simulink model "TST_AirHt_Ctl"  (R2016b)
settings: Solver=FixedStepDiscrete  StartTime=0.0  StopTime=simTime  FixedStep=sampleTime  RelTol=1e-3
values from neighbouring files (symbols this model uses):
  testCase = 1    [initTST_AirHt_Ctl_001.m]    (also in initTST_AirHt_Ctl_002.m = 2; initTST_AirHt_Ctl_003.m = 3; initTST_AirHt_Ctl_004.m = 4; initTST_AirHt_Ctl_005.m = 5)
libraries: simulink x53, UnitTest_Lib x26
(part 3 of 4)

== system TST_AirHt_Ctl/simulationInput/testSignals_R006 ==
  BC : BusCreator  Inputs=21
  spec_AirHt_st : FromWorkspace  VariableName=testSig_AirHt_st  Interpolate=off  OutputAfterFinalValue=Holding final value
  spec_Air_tAFS_mp : FromWorkspace  VariableName=testSig_Air_tAFS_mp  Interpolate=off  OutputAfterFinalValue=Holding final value
  spec_Air_tCACDs_mp : FromWorkspace  VariableName=testSig_Air_tCACDs_mp  Interpolate=off  OutputAfterFinalValue=Holding final value
  spec_Air_tIntkVUs : FromWorkspace  VariableName=testSig_Air_tIntkVUs  Interpolate=off  OutputAfterFinalValue=Holding final value
  spec_BattU_u : FromWorkspace  VariableName=testSig_BattU_u  Interpolate=off  OutputAfterFinalValue=Holding final value
  spec_CEngDsT_t : FromWorkspace  VariableName=testSig_CEngDsT_t  Interpolate=off  OutputAfterFinalValue=Holding final value
  spec_CoEng_st : FromWorkspace  VariableName=testSig_CoEng_st  Interpolate=off  OutputAfterFinalValue=Holding final value
  spec_DSM_bAirHtAFST : FromWorkspace  VariableName=testSig_DSM_bAirHtAFST  Interpolate=off  OutputAfterFinalValue=Holding final value
  spec_DSM_bAirHtCACDs : FromWorkspace  VariableName=testSig_DSM_bAirHtCACDs  Interpolate=off  OutputAfterFinalValue=Holding final value
  spec_DSM_bAirHtCEngDsT : FromWorkspace  VariableName=testSig_DSM_bAirHtCEngDsT  Interpolate=off  OutputAfterFinalValue=Holding final value
  spec_DSM_bAirHtEnvT : FromWorkspace  VariableName=testSig_DSM_bAirHtEnvT  Interpolate=off  OutputAfterFinalValue=Holding final value
  spec_DSM_bAirHtFuelT : FromWorkspace  VariableName=testSig_DSM_bAirHtFuelT  Interpolate=off  OutputAfterFinalValue=Holding final value
  spec_DSM_bAirHtIntkVUsT : FromWorkspace  VariableName=testSig_DSM_bAirHtIntkVUsT  Interpolate=off  OutputAfterFinalValue=Holding final value
  spec_DSM_bAirHtOilT : FromWorkspace  VariableName=testSig_DSM_bAirHtOilT  Interpolate=off  OutputAfterFinalValue=Holding final value
  spec_EnvT_t : FromWorkspace  VariableName=testSig_EnvT_t  Interpolate=off  OutputAfterFinalValue=Holding final value
  spec_Epm_nEng : FromWorkspace  VariableName=testSig_Epm_nEng  Interpolate=off  OutputAfterFinalValue=Holding final value
  spec_FuelT_t : FromWorkspace  VariableName=testSig_FuelT_t  Interpolate=off  OutputAfterFinalValue=Holding final value
  spec_GlwLmp_st : FromWorkspace  VariableName=testSig_GlwLmp_st  Interpolate=off  OutputAfterFinalValue=Holding final value
  spec_IAirHt_st : FromWorkspace  VariableName=testSig_IAirHt_st  Interpolate=off  OutputAfterFinalValue=Holding final value
  spec_Oil_tSwmp : FromWorkspace  VariableName=testSig_Oil_tSwmp  Interpolate=off  OutputAfterFinalValue=Holding final value
  spec_T15_st : FromWorkspace  VariableName=testSig_T15_st  Interpolate=off  OutputAfterFinalValue=Holding final value
  testSignals : Outport
  wires:
  BC/1 -> testSignals/1
  spec_T15_st/1 -> BC/1  "testSig_T15_st"
  spec_CoEng_st/1 -> BC/2  "testSig_CoEng_st"
  spec_Epm_nEng/1 -> BC/3  "testSig_Epm_nEng"
  spec_BattU_u/1 -> BC/4  "testSig_BattU_u"
  spec_CEngDsT_t/1 -> BC/5  "testSig_CEngDsT_t"
  spec_FuelT_t/1 -> BC/6  "testSig_FuelT_t"
  spec_Oil_tSwmp/1 -> BC/7  "testSig_Oil_tSwmp"
  spec_Air_tCACDs_mp/1 -> BC/8  "testSig_Air_tCACDs_mp"
  spec_Air_tAFS_mp/1 -> BC/9  "testSig_Air_tAFS_mp"
  spec_EnvT_t/1 -> BC/10  "testSig_EnvT_t"
  spec_Air_tIntkVUs/1 -> BC/11  "testSig_Air_tIntkVUs"
  spec_DSM_bAirHtCEngDsT/1 -> BC/12  "testSig_DSM_bAirHtCEngDsT"
  spec_DSM_bAirHtFuelT/1 -> BC/13  "testSig_DSM_bAirHtFuelT"
  spec_DSM_bAirHtOilT/1 -> BC/14  "testSig_DSM_bAirHtOilT"
  spec_DSM_bAirHtEnvT/1 -> BC/15  "testSig_DSM_bAirHtEnvT"
  spec_DSM_bAirHtCACDs/1 -> BC/16  "testSig_DSM_bAirHtCACDs"
  spec_DSM_bAirHtAFST/1 -> BC/17  "testSig_DSM_bAirHtAFST"
  spec_DSM_bAirHtIntkVUsT/1 -> BC/18  "testSig_DSM_bAirHtIntkVUsT"
  spec_AirHt_st/1 -> BC/19  "testSig_AirHt_st"
  spec_IAirHt_st/1 -> BC/20  "testSig_IAirHt_st"
  spec_GlwLmp_st/1 -> BC/21  "testSig_GlwLmp_st"

== system TST_AirHt_Ctl/simulationInput/testSignals_R007 ==
  BC : BusCreator  Inputs=21
  spec_AirHt_st : FromWorkspace  VariableName=testSig_AirHt_st  Interpolate=off  OutputAfterFinalValue=Holding final value
  spec_Air_tAFS_mp : FromWorkspace  VariableName=testSig_Air_tAFS_mp  Interpolate=off  OutputAfterFinalValue=Holding final value
  spec_Air_tCACDs_mp : FromWorkspace  VariableName=testSig_Air_tCACDs_mp  Interpolate=off  OutputAfterFinalValue=Holding final value
  spec_Air_tIntkVUs : FromWorkspace  VariableName=testSig_Air_tIntkVUs  Interpolate=off  OutputAfterFinalValue=Holding final value
  spec_BattU_u : FromWorkspace  VariableName=testSig_BattU_u  Interpolate=off  OutputAfterFinalValue=Holding final value
  spec_CEngDsT_t : FromWorkspace  VariableName=testSig_CEngDsT_t  Interpolate=off  OutputAfterFinalValue=Holding final value
  spec_CoEng_st : FromWorkspace  VariableName=testSig_CoEng_st  Interpolate=off  OutputAfterFinalValue=Holding final value
  spec_DSM_bAirHtAFST : FromWorkspace  VariableName=testSig_DSM_bAirHtAFST  Interpolate=off  OutputAfterFinalValue=Holding final value
  spec_DSM_bAirHtCACDs : FromWorkspace  VariableName=testSig_DSM_bAirHtCACDs  Interpolate=off  OutputAfterFinalValue=Holding final value
  spec_DSM_bAirHtCEngDsT : FromWorkspace  VariableName=testSig_DSM_bAirHtCEngDsT  Interpolate=off  OutputAfterFinalValue=Holding final value
  spec_DSM_bAirHtEnvT : FromWorkspace  VariableName=testSig_DSM_bAirHtEnvT  Interpolate=off  OutputAfterFinalValue=Holding final value
  spec_DSM_bAirHtFuelT : FromWorkspace  VariableName=testSig_DSM_bAirHtFuelT  Interpolate=off  OutputAfterFinalValue=Holding final value
  spec_DSM_bAirHtIntkVUsT : FromWorkspace  VariableName=testSig_DSM_bAirHtIntkVUsT  Interpolate=off  OutputAfterFinalValue=Holding final value
  spec_DSM_bAirHtOilT : FromWorkspace  VariableName=testSig_DSM_bAirHtOilT  Interpolate=off  OutputAfterFinalValue=Holding final value
  spec_EnvT_t : FromWorkspace  VariableName=testSig_EnvT_t  Interpolate=off  OutputAfterFinalValue=Holding final value
  spec_Epm_nEng : FromWorkspace  VariableName=testSig_Epm_nEng  Interpolate=off  OutputAfterFinalValue=Holding final value
  spec_FuelT_t : FromWorkspace  VariableName=testSig_FuelT_t  Interpolate=off  OutputAfterFinalValue=Holding final value
  spec_GlwLmp_st : FromWorkspace  VariableName=testSig_GlwLmp_st  Interpolate=off  OutputAfterFinalValue=Holding final value
  spec_IAirHt_st : FromWorkspace  VariableName=testSig_IAirHt_st  Interpolate=off  OutputAfterFinalValue=Holding final value
  spec_Oil_tSwmp : FromWorkspace  VariableName=testSig_Oil_tSwmp  Interpolate=off  OutputAfterFinalValue=Holding final value
  spec_T15_st : FromWorkspace  VariableName=testSig_T15_st  Interpolate=off  OutputAfterFinalValue=Holding final value
  testSignals : Outport
  wires:
  BC/1 -> testSignals/1
  spec_T15_st/1 -> BC/1  "testSig_T15_st"
  spec_CoEng_st/1 -> BC/2  "testSig_CoEng_st"
  spec_Epm_nEng/1 -> BC/3  "testSig_Epm_nEng"
  spec_BattU_u/1 -> BC/4  "testSig_BattU_u"
  spec_CEngDsT_t/1 -> BC/5  "testSig_CEngDsT_t"
  spec_FuelT_t/1 -> BC/6  "testSig_FuelT_t"
  spec_Oil_tSwmp/1 -> BC/7  "testSig_Oil_tSwmp"
  spec_Air_tCACDs_mp/1 -> BC/8  "testSig_Air_tCACDs_mp"
  spec_Air_tAFS_mp/1 -> BC/9  "testSig_Air_tAFS_mp"
  spec_EnvT_t/1 -> BC/10  "testSig_EnvT_t"
  spec_Air_tIntkVUs/1 -> BC/11  "testSig_Air_tIntkVUs"
  spec_DSM_bAirHtCEngDsT/1 -> BC/12  "testSig_DSM_bAirHtCEngDsT"
  spec_DSM_bAirHtFuelT/1 -> BC/13  "testSig_DSM_bAirHtFuelT"
  spec_DSM_bAirHtOilT/1 -> BC/14  "testSig_DSM_bAirHtOilT"
  spec_DSM_bAirHtEnvT/1 -> BC/15  "testSig_DSM_bAirHtEnvT"
  spec_DSM_bAirHtCACDs/1 -> BC/16  "testSig_DSM_bAirHtCACDs"
  spec_DSM_bAirHtAFST/1 -> BC/17  "testSig_DSM_bAirHtAFST"
  spec_DSM_bAirHtIntkVUsT/1 -> BC/18  "testSig_DSM_bAirHtIntkVUsT"
  spec_AirHt_st/1 -> BC/19  "testSig_AirHt_st"
  spec_IAirHt_st/1 -> BC/20  "testSig_IAirHt_st"
  spec_GlwLmp_st/1 -> BC/21  "testSig_GlwLmp_st"

== system TST_AirHt_Ctl/simulationInput/testSignals_R008 ==
  BC : BusCreator  Inputs=21
  spec_AirHt_st : FromWorkspace  VariableName=testSig_AirHt_st  Interpolate=off  OutputAfterFinalValue=Holding final value
  spec_Air_tAFS_mp : FromWorkspace  VariableName=testSig_Air_tAFS_mp  Interpolate=off  OutputAfterFinalValue=Holding final value
  spec_Air_tCACDs_mp : FromWorkspace  VariableName=testSig_Air_tCACDs_mp  Interpolate=off  OutputAfterFinalValue=Holding final value
  spec_Air_tIntkVUs : FromWorkspace  VariableName=testSig_Air_tIntkVUs  Interpolate=off  OutputAfterFinalValue=Holding final value
  spec_BattU_u : FromWorkspace  VariableName=testSig_BattU_u  Interpolate=off  OutputAfterFinalValue=Holding final value
  spec_CEngDsT_t : FromWorkspace  VariableName=testSig_CEngDsT_t  Interpolate=off  OutputAfterFinalValue=Holding final value
  spec_CoEng_st : FromWorkspace  VariableName=testSig_CoEng_st  Interpolate=off  OutputAfterFinalValue=Holding final value
  spec_DSM_bAirHtAFST : FromWorkspace  VariableName=testSig_DSM_bAirHtAFST  Interpolate=off  OutputAfterFinalValue=Holding final value
  spec_DSM_bAirHtCACDs : FromWorkspace  VariableName=testSig_DSM_bAirHtCACDs  Interpolate=off  OutputAfterFinalValue=Holding final value
  spec_DSM_bAirHtCEngDsT : FromWorkspace  VariableName=testSig_DSM_bAirHtCEngDsT  Interpolate=off  OutputAfterFinalValue=Holding final value
  spec_DSM_bAirHtEnvT : FromWorkspace  VariableName=testSig_DSM_bAirHtEnvT  Interpolate=off  OutputAfterFinalValue=Holding final value
  spec_DSM_bAirHtFuelT : FromWorkspace  VariableName=testSig_DSM_bAirHtFuelT  Interpolate=off  OutputAfterFinalValue=Holding final value
  spec_DSM_bAirHtIntkVUsT : FromWorkspace  VariableName=testSig_DSM_bAirHtIntkVUsT  Interpolate=off  OutputAfterFinalValue=Holding final value
  spec_DSM_bAirHtOilT : FromWorkspace  VariableName=testSig_DSM_bAirHtOilT  Interpolate=off  OutputAfterFinalValue=Holding final value
  spec_EnvT_t : FromWorkspace  VariableName=testSig_EnvT_t  Interpolate=off  OutputAfterFinalValue=Holding final value
  spec_Epm_nEng : FromWorkspace  VariableName=testSig_Epm_nEng  Interpolate=off  OutputAfterFinalValue=Holding final value
  spec_FuelT_t : FromWorkspace  VariableName=testSig_FuelT_t  Interpolate=off  OutputAfterFinalValue=Holding final value
  spec_GlwLmp_st : FromWorkspace  VariableName=testSig_GlwLmp_st  Interpolate=off  OutputAfterFinalValue=Holding final value
  spec_IAirHt_st : FromWorkspace  VariableName=testSig_IAirHt_st  Interpolate=off  OutputAfterFinalValue=Holding final value
  spec_Oil_tSwmp : FromWorkspace  VariableName=testSig_Oil_tSwmp  Interpolate=off  OutputAfterFinalValue=Holding final value
  spec_T15_st : FromWorkspace  VariableName=testSig_T15_st  Interpolate=off  OutputAfterFinalValue=Holding final value
  testSignals : Outport
  wires:
  BC/1 -> testSignals/1
  spec_T15_st/1 -> BC/1  "testSig_T15_st"
  spec_CoEng_st/1 -> BC/2  "testSig_CoEng_st"
  spec_Epm_nEng/1 -> BC/3  "testSig_Epm_nEng"
  spec_BattU_u/1 -> BC/4  "testSig_BattU_u"
  spec_CEngDsT_t/1 -> BC/5  "testSig_CEngDsT_t"
  spec_FuelT_t/1 -> BC/6  "testSig_FuelT_t"
  spec_Oil_tSwmp/1 -> BC/7  "testSig_Oil_tSwmp"
  spec_Air_tCACDs_mp/1 -> BC/8  "testSig_Air_tCACDs_mp"
  spec_Air_tAFS_mp/1 -> BC/9  "testSig_Air_tAFS_mp"
  spec_EnvT_t/1 -> BC/10  "testSig_EnvT_t"
  spec_Air_tIntkVUs/1 -> BC/11  "testSig_Air_tIntkVUs"
  spec_DSM_bAirHtCEngDsT/1 -> BC/12  "testSig_DSM_bAirHtCEngDsT"
  spec_DSM_bAirHtFuelT/1 -> BC/13  "testSig_DSM_bAirHtFuelT"
  spec_DSM_bAirHtOilT/1 -> BC/14  "testSig_DSM_bAirHtOilT"
  spec_DSM_bAirHtEnvT/1 -> BC/15  "testSig_DSM_bAirHtEnvT"
  spec_DSM_bAirHtCACDs/1 -> BC/16  "testSig_DSM_bAirHtCACDs"
  spec_DSM_bAirHtAFST/1 -> BC/17  "testSig_DSM_bAirHtAFST"
  spec_DSM_bAirHtIntkVUsT/1 -> BC/18  "testSig_DSM_bAirHtIntkVUsT"
  spec_AirHt_st/1 -> BC/19  "testSig_AirHt_st"
  spec_IAirHt_st/1 -> BC/20  "testSig_IAirHt_st"
  spec_GlwLmp_st/1 -> BC/21  "testSig_GlwLmp_st"

== system TST_AirHt_Ctl/simulationInput/testSignals_R009 ==
  BC : BusCreator  Inputs=21
  spec_AirHt_st : FromWorkspace  VariableName=testSig_AirHt_st  Interpolate=off  OutputAfterFinalValue=Holding final value
  spec_Air_tAFS_mp : FromWorkspace  VariableName=testSig_Air_tAFS_mp  Interpolate=off  OutputAfterFinalValue=Holding final value
  spec_Air_tCACDs_mp : FromWorkspace  VariableName=testSig_Air_tCACDs_mp  Interpolate=off  OutputAfterFinalValue=Holding final value
  spec_Air_tIntkVUs : FromWorkspace  VariableName=testSig_Air_tIntkVUs  Interpolate=off  OutputAfterFinalValue=Holding final value
  spec_BattU_u : FromWorkspace  VariableName=testSig_BattU_u  Interpolate=off  OutputAfterFinalValue=Holding final value
  spec_CEngDsT_t : FromWorkspace  VariableName=testSig_CEngDsT_t  Interpolate=off  OutputAfterFinalValue=Holding final value
  spec_CoEng_st : FromWorkspace  VariableName=testSig_CoEng_st  Interpolate=off  OutputAfterFinalValue=Holding final value
  spec_DSM_bAirHtAFST : FromWorkspace  VariableName=testSig_DSM_bAirHtAFST  Interpolate=off  OutputAfterFinalValue=Holding final value
  spec_DSM_bAirHtCACDs : FromWorkspace  VariableName=testSig_DSM_bAirHtCACDs  Interpolate=off  OutputAfterFinalValue=Holding final value
  spec_DSM_bAirHtCEngDsT : FromWorkspace  VariableName=testSig_DSM_bAirHtCEngDsT  Interpolate=off  OutputAfterFinalValue=Holding final value
  spec_DSM_bAirHtEnvT : FromWorkspace  VariableName=testSig_DSM_bAirHtEnvT  Interpolate=off  OutputAfterFinalValue=Holding final value
  spec_DSM_bAirHtFuelT : FromWorkspace  VariableName=testSig_DSM_bAirHtFuelT  Interpolate=off  OutputAfterFinalValue=Holding final value
  spec_DSM_bAirHtIntkVUsT : FromWorkspace  VariableName=testSig_DSM_bAirHtIntkVUsT  Interpolate=off  OutputAfterFinalValue=Holding final value
  spec_DSM_bAirHtOilT : FromWorkspace  VariableName=testSig_DSM_bAirHtOilT  Interpolate=off  OutputAfterFinalValue=Holding final value
  spec_EnvT_t : FromWorkspace  VariableName=testSig_EnvT_t  Interpolate=off  OutputAfterFinalValue=Holding final value
  spec_Epm_nEng : FromWorkspace  VariableName=testSig_Epm_nEng  Interpolate=off  OutputAfterFinalValue=Holding final value
  spec_FuelT_t : FromWorkspace  VariableName=testSig_FuelT_t  Interpolate=off  OutputAfterFinalValue=Holding final value
  spec_GlwLmp_st : FromWorkspace  VariableName=testSig_GlwLmp_st  Interpolate=off  OutputAfterFinalValue=Holding final value
  spec_IAirHt_st : FromWorkspace  VariableName=testSig_IAirHt_st  Interpolate=off  OutputAfterFinalValue=Holding final value
  spec_Oil_tSwmp : FromWorkspace  VariableName=testSig_Oil_tSwmp  Interpolate=off  OutputAfterFinalValue=Holding final value
  spec_T15_st : FromWorkspace  VariableName=testSig_T15_st  Interpolate=off  OutputAfterFinalValue=Holding final value
  testSignals : Outport
  wires:
  BC/1 -> testSignals/1
  spec_T15_st/1 -> BC/1  "testSig_T15_st"
  spec_CoEng_st/1 -> BC/2  "testSig_CoEng_st"
  spec_Epm_nEng/1 -> BC/3  "testSig_Epm_nEng"
  spec_BattU_u/1 -> BC/4  "testSig_BattU_u"
  spec_CEngDsT_t/1 -> BC/5  "testSig_CEngDsT_t"
  spec_FuelT_t/1 -> BC/6  "testSig_FuelT_t"
  spec_Oil_tSwmp/1 -> BC/7  "testSig_Oil_tSwmp"
  spec_Air_tCACDs_mp/1 -> BC/8  "testSig_Air_tCACDs_mp"
  spec_Air_tAFS_mp/1 -> BC/9  "testSig_Air_tAFS_mp"
  spec_EnvT_t/1 -> BC/10  "testSig_EnvT_t"
  spec_Air_tIntkVUs/1 -> BC/11  "testSig_Air_tIntkVUs"
  spec_DSM_bAirHtCEngDsT/1 -> BC/12  "testSig_DSM_bAirHtCEngDsT"
  spec_DSM_bAirHtFuelT/1 -> BC/13  "testSig_DSM_bAirHtFuelT"
  spec_DSM_bAirHtOilT/1 -> BC/14  "testSig_DSM_bAirHtOilT"
  spec_DSM_bAirHtEnvT/1 -> BC/15  "testSig_DSM_bAirHtEnvT"
  spec_DSM_bAirHtCACDs/1 -> BC/16  "testSig_DSM_bAirHtCACDs"
  spec_DSM_bAirHtAFST/1 -> BC/17  "testSig_DSM_bAirHtAFST"
  spec_DSM_bAirHtIntkVUsT/1 -> BC/18  "testSig_DSM_bAirHtIntkVUsT"
  spec_AirHt_st/1 -> BC/19  "testSig_AirHt_st"
  spec_IAirHt_st/1 -> BC/20  "testSig_IAirHt_st"
  spec_GlwLmp_st/1 -> BC/21  "testSig_GlwLmp_st"

== system TST_AirHt_Ctl/simulationInput/testSignals_R010 ==
  BC : BusCreator  Inputs=21
  spec_AirHt_st : FromWorkspace  VariableName=testSig_AirHt_st  Interpolate=off  OutputAfterFinalValue=Holding final value
  spec_Air_tAFS_mp : FromWorkspace  VariableName=testSig_Air_tAFS_mp  Interpolate=off  OutputAfterFinalValue=Holding final value
  spec_Air_tCACDs_mp : FromWorkspace  VariableName=testSig_Air_tCACDs_mp  Interpolate=off  OutputAfterFinalValue=Holding final value
  spec_Air_tIntkVUs : FromWorkspace  VariableName=testSig_Air_tIntkVUs  Interpolate=off  OutputAfterFinalValue=Holding final value
  spec_BattU_u : FromWorkspace  VariableName=testSig_BattU_u  Interpolate=off  OutputAfterFinalValue=Holding final value
  spec_CEngDsT_t : FromWorkspace  VariableName=testSig_CEngDsT_t  Interpolate=off  OutputAfterFinalValue=Holding final value
  spec_CoEng_st : FromWorkspace  VariableName=testSig_CoEng_st  Interpolate=off  OutputAfterFinalValue=Holding final value
  spec_DSM_bAirHtAFST : FromWorkspace  VariableName=testSig_DSM_bAirHtAFST  Interpolate=off  OutputAfterFinalValue=Holding final value
  spec_DSM_bAirHtCACDs : FromWorkspace  VariableName=testSig_DSM_bAirHtCACDs  Interpolate=off  OutputAfterFinalValue=Holding final value
  spec_DSM_bAirHtCEngDsT : FromWorkspace  VariableName=testSig_DSM_bAirHtCEngDsT  Interpolate=off  OutputAfterFinalValue=Holding final value
  spec_DSM_bAirHtEnvT : FromWorkspace  VariableName=testSig_DSM_bAirHtEnvT  Interpolate=off  OutputAfterFinalValue=Holding final value
  spec_DSM_bAirHtFuelT : FromWorkspace  VariableName=testSig_DSM_bAirHtFuelT  Interpolate=off  OutputAfterFinalValue=Holding final value
  spec_DSM_bAirHtIntkVUsT : FromWorkspace  VariableName=testSig_DSM_bAirHtIntkVUsT  Interpolate=off  OutputAfterFinalValue=Holding final value
  spec_DSM_bAirHtOilT : FromWorkspace  VariableName=testSig_DSM_bAirHtOilT  Interpolate=off  OutputAfterFinalValue=Holding final value
  spec_EnvT_t : FromWorkspace  VariableName=testSig_EnvT_t  Interpolate=off  OutputAfterFinalValue=Holding final value
  spec_Epm_nEng : FromWorkspace  VariableName=testSig_Epm_nEng  Interpolate=off  OutputAfterFinalValue=Holding final value
  spec_FuelT_t : FromWorkspace  VariableName=testSig_FuelT_t  Interpolate=off  OutputAfterFinalValue=Holding final value
  spec_GlwLmp_st : FromWorkspace  VariableName=testSig_GlwLmp_st  Interpolate=off  OutputAfterFinalValue=Holding final value
  spec_IAirHt_st : FromWorkspace  VariableName=testSig_IAirHt_st  Interpolate=off  OutputAfterFinalValue=Holding final value
  spec_Oil_tSwmp : FromWorkspace  VariableName=testSig_Oil_tSwmp  Interpolate=off  OutputAfterFinalValue=Holding final value
  spec_T15_st : FromWorkspace  VariableName=testSig_T15_st  Interpolate=off  OutputAfterFinalValue=Holding final value
  testSignals : Outport
  wires:
  BC/1 -> testSignals/1
  spec_T15_st/1 -> BC/1  "testSig_T15_st"
  spec_CoEng_st/1 -> BC/2  "testSig_CoEng_st"
  spec_Epm_nEng/1 -> BC/3  "testSig_Epm_nEng"
  spec_BattU_u/1 -> BC/4  "testSig_BattU_u"
  spec_CEngDsT_t/1 -> BC/5  "testSig_CEngDsT_t"
  spec_FuelT_t/1 -> BC/6  "testSig_FuelT_t"
  spec_Oil_tSwmp/1 -> BC/7  "testSig_Oil_tSwmp"
  spec_Air_tCACDs_mp/1 -> BC/8  "testSig_Air_tCACDs_mp"
  spec_Air_tAFS_mp/1 -> BC/9  "testSig_Air_tAFS_mp"
  spec_EnvT_t/1 -> BC/10  "testSig_EnvT_t"
  spec_Air_tIntkVUs/1 -> BC/11  "testSig_Air_tIntkVUs"
  spec_DSM_bAirHtCEngDsT/1 -> BC/12  "testSig_DSM_bAirHtCEngDsT"
  spec_DSM_bAirHtFuelT/1 -> BC/13  "testSig_DSM_bAirHtFuelT"
  spec_DSM_bAirHtOilT/1 -> BC/14  "testSig_DSM_bAirHtOilT"
  spec_DSM_bAirHtEnvT/1 -> BC/15  "testSig_DSM_bAirHtEnvT"
  spec_DSM_bAirHtCACDs/1 -> BC/16  "testSig_DSM_bAirHtCACDs"
  spec_DSM_bAirHtAFST/1 -> BC/17  "testSig_DSM_bAirHtAFST"
  spec_DSM_bAirHtIntkVUsT/1 -> BC/18  "testSig_DSM_bAirHtIntkVUsT"
  spec_AirHt_st/1 -> BC/19  "testSig_AirHt_st"
  spec_IAirHt_st/1 -> BC/20  "testSig_IAirHt_st"
  spec_GlwLmp_st/1 -> BC/21  "testSig_GlwLmp_st"

== system TST_AirHt_Ctl/simulationInput/testSignals_R011 ==
  BC : BusCreator  Inputs=21
  spec_AirHt_st : FromWorkspace  VariableName=testSig_AirHt_st  Interpolate=off  OutputAfterFinalValue=Holding final value
  spec_Air_tAFS_mp : FromWorkspace  VariableName=testSig_Air_tAFS_mp  Interpolate=off  OutputAfterFinalValue=Holding final value
  spec_Air_tCACDs_mp : FromWorkspace  VariableName=testSig_Air_tCACDs_mp  Interpolate=off  OutputAfterFinalValue=Holding final value
  spec_Air_tIntkVUs : FromWorkspace  VariableName=testSig_Air_tIntkVUs  Interpolate=off  OutputAfterFinalValue=Holding final value
  spec_BattU_u : FromWorkspace  VariableName=testSig_BattU_u  Interpolate=off  OutputAfterFinalValue=Holding final value
  spec_CEngDsT_t : FromWorkspace  VariableName=testSig_CEngDsT_t  Interpolate=off  OutputAfterFinalValue=Holding final value
  spec_CoEng_st : FromWorkspace  VariableName=testSig_CoEng_st  Interpolate=off  OutputAfterFinalValue=Holding final value
  spec_DSM_bAirHtAFST : FromWorkspace  VariableName=testSig_DSM_bAirHtAFST  Interpolate=off  OutputAfterFinalValue=Holding final value
  spec_DSM_bAirHtCACDs : FromWorkspace  VariableName=testSig_DSM_bAirHtCACDs  Interpolate=off  OutputAfterFinalValue=Holding final value
  spec_DSM_bAirHtCEngDsT : FromWorkspace  VariableName=testSig_DSM_bAirHtCEngDsT  Interpolate=off  OutputAfterFinalValue=Holding final value
  spec_DSM_bAirHtEnvT : FromWorkspace  VariableName=testSig_DSM_bAirHtEnvT  Interpolate=off  OutputAfterFinalValue=Holding final value
  spec_DSM_bAirHtFuelT : FromWorkspace  VariableName=testSig_DSM_bAirHtFuelT  Interpolate=off  OutputAfterFinalValue=Holding final value
  spec_DSM_bAirHtIntkVUsT : FromWorkspace  VariableName=testSig_DSM_bAirHtIntkVUsT  Interpolate=off  OutputAfterFinalValue=Holding final value
  spec_DSM_bAirHtOilT : FromWorkspace  VariableName=testSig_DSM_bAirHtOilT  Interpolate=off  OutputAfterFinalValue=Holding final value
  spec_EnvT_t : FromWorkspace  VariableName=testSig_EnvT_t  Interpolate=off  OutputAfterFinalValue=Holding final value
  spec_Epm_nEng : FromWorkspace  VariableName=testSig_Epm_nEng  Interpolate=off  OutputAfterFinalValue=Holding final value
  spec_FuelT_t : FromWorkspace  VariableName=testSig_FuelT_t  Interpolate=off  OutputAfterFinalValue=Holding final value
  spec_GlwLmp_st : FromWorkspace  VariableName=testSig_GlwLmp_st  Interpolate=off  OutputAfterFinalValue=Holding final value
  spec_IAirHt_st : FromWorkspace  VariableName=testSig_IAirHt_st  Interpolate=off  OutputAfterFinalValue=Holding final value
  spec_Oil_tSwmp : FromWorkspace  VariableName=testSig_Oil_tSwmp  Interpolate=off  OutputAfterFinalValue=Holding final value
  spec_T15_st : FromWorkspace  VariableName=testSig_T15_st  Interpolate=off  OutputAfterFinalValue=Holding final value
  testSignals : Outport
  wires:
  BC/1 -> testSignals/1
  spec_T15_st/1 -> BC/1  "testSig_T15_st"
  spec_CoEng_st/1 -> BC/2  "testSig_CoEng_st"
  spec_Epm_nEng/1 -> BC/3  "testSig_Epm_nEng"
  spec_BattU_u/1 -> BC/4  "testSig_BattU_u"
  spec_CEngDsT_t/1 -> BC/5  "testSig_CEngDsT_t"
  spec_FuelT_t/1 -> BC/6  "testSig_FuelT_t"
  spec_Oil_tSwmp/1 -> BC/7  "testSig_Oil_tSwmp"
  spec_Air_tCACDs_mp/1 -> BC/8  "testSig_Air_tCACDs_mp"
  spec_Air_tAFS_mp/1 -> BC/9  "testSig_Air_tAFS_mp"
  spec_EnvT_t/1 -> BC/10  "testSig_EnvT_t"
  spec_Air_tIntkVUs/1 -> BC/11  "testSig_Air_tIntkVUs"
  spec_DSM_bAirHtCEngDsT/1 -> BC/12  "testSig_DSM_bAirHtCEngDsT"
  spec_DSM_bAirHtFuelT/1 -> BC/13  "testSig_DSM_bAirHtFuelT"
  spec_DSM_bAirHtOilT/1 -> BC/14  "testSig_DSM_bAirHtOilT"
  spec_DSM_bAirHtEnvT/1 -> BC/15  "testSig_DSM_bAirHtEnvT"
  spec_DSM_bAirHtCACDs/1 -> BC/16  "testSig_DSM_bAirHtCACDs"
  spec_DSM_bAirHtAFST/1 -> BC/17  "testSig_DSM_bAirHtAFST"
  spec_DSM_bAirHtIntkVUsT/1 -> BC/18  "testSig_DSM_bAirHtIntkVUsT"
  spec_AirHt_st/1 -> BC/19  "testSig_AirHt_st"
  spec_IAirHt_st/1 -> BC/20  "testSig_IAirHt_st"
  spec_GlwLmp_st/1 -> BC/21  "testSig_GlwLmp_st"

== system TST_AirHt_Ctl/simulationInput/testSignals_R012 ==
  BC : BusCreator  Inputs=21
  spec_AirHt_st : FromWorkspace  VariableName=testSig_AirHt_st  Interpolate=off  OutputAfterFinalValue=Holding final value
  spec_Air_tAFS_mp : FromWorkspace  VariableName=testSig_Air_tAFS_mp  Interpolate=off  OutputAfterFinalValue=Holding final value
  spec_Air_tCACDs_mp : FromWorkspace  VariableName=testSig_Air_tCACDs_mp  Interpolate=off  OutputAfterFinalValue=Holding final value
  spec_Air_tIntkVUs : FromWorkspace  VariableName=testSig_Air_tIntkVUs  Interpolate=off  OutputAfterFinalValue=Holding final value
  spec_BattU_u : FromWorkspace  VariableName=testSig_BattU_u  Interpolate=off  OutputAfterFinalValue=Holding final value
  spec_CEngDsT_t : FromWorkspace  VariableName=testSig_CEngDsT_t  Interpolate=off  OutputAfterFinalValue=Holding final value
  spec_CoEng_st : FromWorkspace  VariableName=testSig_CoEng_st  Interpolate=off  OutputAfterFinalValue=Holding final value
  spec_DSM_bAirHtAFST : FromWorkspace  VariableName=testSig_DSM_bAirHtAFST  Interpolate=off  OutputAfterFinalValue=Holding final value
  spec_DSM_bAirHtCACDs : FromWorkspace  VariableName=testSig_DSM_bAirHtCACDs  Interpolate=off  OutputAfterFinalValue=Holding final value
  spec_DSM_bAirHtCEngDsT : FromWorkspace  VariableName=testSig_DSM_bAirHtCEngDsT  Interpolate=off  OutputAfterFinalValue=Holding final value
  spec_DSM_bAirHtEnvT : FromWorkspace  VariableName=testSig_DSM_bAirHtEnvT  Interpolate=off  OutputAfterFinalValue=Holding final value
  spec_DSM_bAirHtFuelT : FromWorkspace  VariableName=testSig_DSM_bAirHtFuelT  Interpolate=off  OutputAfterFinalValue=Holding final value
  spec_DSM_bAirHtIntkVUsT : FromWorkspace  VariableName=testSig_DSM_bAirHtIntkVUsT  Interpolate=off  OutputAfterFinalValue=Holding final value
  spec_DSM_bAirHtOilT : FromWorkspace  VariableName=testSig_DSM_bAirHtOilT  Interpolate=off  OutputAfterFinalValue=Holding final value
  spec_EnvT_t : FromWorkspace  VariableName=testSig_EnvT_t  Interpolate=off  OutputAfterFinalValue=Holding final value
  spec_Epm_nEng : FromWorkspace  VariableName=testSig_Epm_nEng  Interpolate=off  OutputAfterFinalValue=Holding final value
  spec_FuelT_t : FromWorkspace  VariableName=testSig_FuelT_t  Interpolate=off  OutputAfterFinalValue=Holding final value
  spec_GlwLmp_st : FromWorkspace  VariableName=testSig_GlwLmp_st  Interpolate=off  OutputAfterFinalValue=Holding final value
  spec_IAirHt_st : FromWorkspace  VariableName=testSig_IAirHt_st  Interpolate=off  OutputAfterFinalValue=Holding final value
  spec_Oil_tSwmp : FromWorkspace  VariableName=testSig_Oil_tSwmp  Interpolate=off  OutputAfterFinalValue=Holding final value
  spec_T15_st : FromWorkspace  VariableName=testSig_T15_st  Interpolate=off  OutputAfterFinalValue=Holding final value
  testSignals : Outport
  wires:
  BC/1 -> testSignals/1
  spec_T15_st/1 -> BC/1  "testSig_T15_st"
  spec_CoEng_st/1 -> BC/2  "testSig_CoEng_st"
  spec_Epm_nEng/1 -> BC/3  "testSig_Epm_nEng"
  spec_BattU_u/1 -> BC/4  "testSig_BattU_u"
  spec_CEngDsT_t/1 -> BC/5  "testSig_CEngDsT_t"
  spec_FuelT_t/1 -> BC/6  "testSig_FuelT_t"
  spec_Oil_tSwmp/1 -> BC/7  "testSig_Oil_tSwmp"
  spec_Air_tCACDs_mp/1 -> BC/8  "testSig_Air_tCACDs_mp"
  spec_Air_tAFS_mp/1 -> BC/9  "testSig_Air_tAFS_mp"
  spec_EnvT_t/1 -> BC/10  "testSig_EnvT_t"
  spec_Air_tIntkVUs/1 -> BC/11  "testSig_Air_tIntkVUs"
  spec_DSM_bAirHtCEngDsT/1 -> BC/12  "testSig_DSM_bAirHtCEngDsT"
  spec_DSM_bAirHtFuelT/1 -> BC/13  "testSig_DSM_bAirHtFuelT"
  spec_DSM_bAirHtOilT/1 -> BC/14  "testSig_DSM_bAirHtOilT"
  spec_DSM_bAirHtEnvT/1 -> BC/15  "testSig_DSM_bAirHtEnvT"
  spec_DSM_bAirHtCACDs/1 -> BC/16  "testSig_DSM_bAirHtCACDs"
  spec_DSM_bAirHtAFST/1 -> BC/17  "testSig_DSM_bAirHtAFST"
  spec_DSM_bAirHtIntkVUsT/1 -> BC/18  "testSig_DSM_bAirHtIntkVUsT"
  spec_AirHt_st/1 -> BC/19  "testSig_AirHt_st"
  spec_IAirHt_st/1 -> BC/20  "testSig_IAirHt_st"
  spec_GlwLmp_st/1 -> BC/21  "testSig_GlwLmp_st"

== system TST_AirHt_Ctl/simulationInput/testSignals_R013 ==
  BC : BusCreator  Inputs=21
  spec_AirHt_st : FromWorkspace  VariableName=testSig_AirHt_st  Interpolate=off  OutputAfterFinalValue=Holding final value
  spec_Air_tAFS_mp : FromWorkspace  VariableName=testSig_Air_tAFS_mp  Interpolate=off  OutputAfterFinalValue=Holding final value
  spec_Air_tCACDs_mp : FromWorkspace  VariableName=testSig_Air_tCACDs_mp  Interpolate=off  OutputAfterFinalValue=Holding final value
  spec_Air_tIntkVUs : FromWorkspace  VariableName=testSig_Air_tIntkVUs  Interpolate=off  OutputAfterFinalValue=Holding final value
  spec_BattU_u : FromWorkspace  VariableName=testSig_BattU_u  Interpolate=off  OutputAfterFinalValue=Holding final value
  spec_CEngDsT_t : FromWorkspace  VariableName=testSig_CEngDsT_t  Interpolate=off  OutputAfterFinalValue=Holding final value
  spec_CoEng_st : FromWorkspace  VariableName=testSig_CoEng_st  Interpolate=off  OutputAfterFinalValue=Holding final value
  spec_DSM_bAirHtAFST : FromWorkspace  VariableName=testSig_DSM_bAirHtAFST  Interpolate=off  OutputAfterFinalValue=Holding final value
  spec_DSM_bAirHtCACDs : FromWorkspace  VariableName=testSig_DSM_bAirHtCACDs  Interpolate=off  OutputAfterFinalValue=Holding final value
  spec_DSM_bAirHtCEngDsT : FromWorkspace  VariableName=testSig_DSM_bAirHtCEngDsT  Interpolate=off  OutputAfterFinalValue=Holding final value
  spec_DSM_bAirHtEnvT : FromWorkspace  VariableName=testSig_DSM_bAirHtEnvT  Interpolate=off  OutputAfterFinalValue=Holding final value
  spec_DSM_bAirHtFuelT : FromWorkspace  VariableName=testSig_DSM_bAirHtFuelT  Interpolate=off  OutputAfterFinalValue=Holding final value
  spec_DSM_bAirHtIntkVUsT : FromWorkspace  VariableName=testSig_DSM_bAirHtIntkVUsT  Interpolate=off  OutputAfterFinalValue=Holding final value
  spec_DSM_bAirHtOilT : FromWorkspace  VariableName=testSig_DSM_bAirHtOilT  Interpolate=off  OutputAfterFinalValue=Holding final value
  spec_EnvT_t : FromWorkspace  VariableName=testSig_EnvT_t  Interpolate=off  OutputAfterFinalValue=Holding final value
  spec_Epm_nEng : FromWorkspace  VariableName=testSig_Epm_nEng  Interpolate=off  OutputAfterFinalValue=Holding final value
  spec_FuelT_t : FromWorkspace  VariableName=testSig_FuelT_t  Interpolate=off  OutputAfterFinalValue=Holding final value
  spec_GlwLmp_st : FromWorkspace  VariableName=testSig_GlwLmp_st  Interpolate=off  OutputAfterFinalValue=Holding final value
  spec_IAirHt_st : FromWorkspace  VariableName=testSig_IAirHt_st  Interpolate=off  OutputAfterFinalValue=Holding final value
  spec_Oil_tSwmp : FromWorkspace  VariableName=testSig_Oil_tSwmp  Interpolate=off  OutputAfterFinalValue=Holding final value
  spec_T15_st : FromWorkspace  VariableName=testSig_T15_st  Interpolate=off  OutputAfterFinalValue=Holding final value
  testSignals : Outport
  wires:
  BC/1 -> testSignals/1
  spec_T15_st/1 -> BC/1  "testSig_T15_st"
  spec_CoEng_st/1 -> BC/2  "testSig_CoEng_st"
  spec_Epm_nEng/1 -> BC/3  "testSig_Epm_nEng"
  spec_BattU_u/1 -> BC/4  "testSig_BattU_u"
  spec_CEngDsT_t/1 -> BC/5  "testSig_CEngDsT_t"
  spec_FuelT_t/1 -> BC/6  "testSig_FuelT_t"
  spec_Oil_tSwmp/1 -> BC/7  "testSig_Oil_tSwmp"
  spec_Air_tCACDs_mp/1 -> BC/8  "testSig_Air_tCACDs_mp"
  spec_Air_tAFS_mp/1 -> BC/9  "testSig_Air_tAFS_mp"
  spec_EnvT_t/1 -> BC/10  "testSig_EnvT_t"
  spec_Air_tIntkVUs/1 -> BC/11  "testSig_Air_tIntkVUs"
  spec_DSM_bAirHtCEngDsT/1 -> BC/12  "testSig_DSM_bAirHtCEngDsT"
  spec_DSM_bAirHtFuelT/1 -> BC/13  "testSig_DSM_bAirHtFuelT"
  spec_DSM_bAirHtOilT/1 -> BC/14  "testSig_DSM_bAirHtOilT"
  spec_DSM_bAirHtEnvT/1 -> BC/15  "testSig_DSM_bAirHtEnvT"
  spec_DSM_bAirHtCACDs/1 -> BC/16  "testSig_DSM_bAirHtCACDs"
  spec_DSM_bAirHtAFST/1 -> BC/17  "testSig_DSM_bAirHtAFST"
  spec_DSM_bAirHtIntkVUsT/1 -> BC/18  "testSig_DSM_bAirHtIntkVUsT"
  spec_AirHt_st/1 -> BC/19  "testSig_AirHt_st"
  spec_IAirHt_st/1 -> BC/20  "testSig_IAirHt_st"
  spec_GlwLmp_st/1 -> BC/21  "testSig_GlwLmp_st"

== system TST_AirHt_Ctl/compareSignals/Requirement_001/specifyOutputs ==
  sig_Req_Bus : Inport
  sig_Result_Bus : Inport  Port=2
  AndN : Logic  Inputs=3
  BS_Req : BusSelector  OutputSignals=testSig_AirHt_st,testSig_IAirHt_st,testSig_GlwLmp_st
  BS_Result : BusSelector  OutputSignals=AirHt_st,IAirHt_st,GlwLmp_st
  Bitwise_And1 : simulink/Logic and Bit Operations/Bitwise Operator  logicop=AND  UseBitMask=off  BitMask=bin2dec('11011001')  BitMaskRealWorld=Stored Integer
  Bitwise_And2 : simulink/Logic and Bit Operations/Bitwise Operator  logicop=AND  UseBitMask=off  BitMask=bin2dec('11011001')  BitMaskRealWorld=Stored Integer
  Bitwise_And3 : simulink/Logic and Bit Operations/Bitwise Operator  logicop=AND  UseBitMask=off  BitMask=bin2dec('11011001')  BitMaskRealWorld=Stored Integer
  Relational Operator : RelationalOperator  Operator===  OutDataTypeStr=boolean  RndMeth=Simplest
  Scope : Scope  NumInputPorts=3
  Scope1 : Scope  NumInputPorts=2
  Scope2 : Scope  NumInputPorts=2
  Scope3 : Scope  NumInputPorts=2
  cmp_2 : UnitTest_Lib/RoughlyEqual  slope=0.1
  cmp_3 : UnitTest_Lib/RoughlyEqual  slope=0.1
  result_tws : ToWorkspace  VariableName=spec_result_001
  tws_1 : ToWorkspace  VariableName=spec_req_001_001
  tws_2 : ToWorkspace  VariableName=spec_req_001_002
  tws_3 : ToWorkspace  VariableName=spec_req_001_003
  result : Outport
  wires:
  sig_Req_Bus/1 -> BS_Req/1
  sig_Result_Bus/1 -> BS_Result/1
  AndN/1 -> result/1, result_tws/1
  BS_Req/1 -> Relational Operator/1, Scope1/1  "<testSig_AirHt_st>"
  BS_Result/1 -> Relational Operator/2, Scope1/2  "<AirHt_st>"
  Relational Operator/1 -> Bitwise_And1/1
  Bitwise_And1/1 -> AndN/1, Scope/1, tws_1/1
  BS_Req/2 -> cmp_2/1, Scope2/1  "<testSig_IAirHt_st>"
  BS_Result/2 -> cmp_2/2, Scope2/2  "<IAirHt_st>"
  cmp_2/1 -> Bitwise_And2/1
  Bitwise_And2/1 -> AndN/2, Scope/2, tws_2/1
  BS_Req/3 -> cmp_3/1, Scope3/1  "<testSig_GlwLmp_st>"
  BS_Result/3 -> cmp_3/2, Scope3/2  "<GlwLmp_st>"
  cmp_3/1 -> Bitwise_And3/1
  Bitwise_And3/1 -> AndN/3, Scope/3, tws_3/1

== system TST_AirHt_Ctl/compareSignals/Requirement_002/specifyOutputs ==
  sig_Req_Bus : Inport
  sig_Result_Bus : Inport  Port=2
  AndN : Logic  Inputs=3
  BS_Req : BusSelector  OutputSignals=testSig_AirHt_st,testSig_IAirHt_st,testSig_GlwLmp_st
  BS_Result : BusSelector  OutputSignals=AirHt_st,IAirHt_st,GlwLmp_st
  Bitwise_And1 : simulink/Logic and Bit Operations/Bitwise Operator  logicop=AND  UseBitMask=off  BitMask=bin2dec('11011001')  BitMaskRealWorld=Stored Integer
  Bitwise_And2 : simulink/Logic and Bit Operations/Bitwise Operator  logicop=AND  UseBitMask=off  BitMask=bin2dec('11011001')  BitMaskRealWorld=Stored Integer
  Bitwise_And3 : simulink/Logic and Bit Operations/Bitwise Operator  logicop=AND  UseBitMask=off  BitMask=bin2dec('11011001')  BitMaskRealWorld=Stored Integer
  Relational Operator : RelationalOperator  Operator===  OutDataTypeStr=boolean  RndMeth=Simplest
  Scope : Scope  NumInputPorts=3
  Scope1 : Scope  NumInputPorts=2
  Scope2 : Scope  NumInputPorts=2
  Scope3 : Scope  NumInputPorts=2
  cmp_2 : UnitTest_Lib/RoughlyEqual  slope=0.1
  cmp_3 : UnitTest_Lib/RoughlyEqual  slope=0.1
  result_tws : ToWorkspace  VariableName=spec_result_002
  tws_1 : ToWorkspace  VariableName=spec_req_002_001
  tws_2 : ToWorkspace  VariableName=spec_req_002_002
  tws_3 : ToWorkspace  VariableName=spec_req_002_003
  result : Outport
  wires:
  sig_Req_Bus/1 -> BS_Req/1
  sig_Result_Bus/1 -> BS_Result/1
  AndN/1 -> result/1, result_tws/1
  BS_Req/1 -> Relational Operator/1, Scope1/1  "<testSig_AirHt_st>"
  BS_Result/1 -> Relational Operator/2, Scope1/2  "<AirHt_st>"
  Relational Operator/1 -> Bitwise_And1/1
  Bitwise_And1/1 -> AndN/1, Scope/1, tws_1/1
  BS_Req/2 -> cmp_2/1, Scope2/1  "<testSig_IAirHt_st>"
  BS_Result/2 -> cmp_2/2, Scope2/2  "<IAirHt_st>"
  cmp_2/1 -> Bitwise_And2/1
  Bitwise_And2/1 -> AndN/2, Scope/2, tws_2/1
  BS_Req/3 -> cmp_3/1, Scope3/1  "<testSig_GlwLmp_st>"
  BS_Result/3 -> cmp_3/2, Scope3/2  "<GlwLmp_st>"
  cmp_3/1 -> Bitwise_And3/1
  Bitwise_And3/1 -> AndN/3, Scope/3, tws_3/1

== system TST_AirHt_Ctl/compareSignals/Requirement_003/specifyOutputs ==
  sig_Req_Bus : Inport
  sig_Result_Bus : Inport  Port=2
  AndN : Logic  Inputs=3
  BS_Req : BusSelector  OutputSignals=testSig_AirHt_st,testSig_IAirHt_st,testSig_GlwLmp_st
  BS_Result : BusSelector  OutputSignals=AirHt_st,IAirHt_st,GlwLmp_st
  Bitwise_And1 : simulink/Logic and Bit Operations/Bitwise Operator  logicop=AND  UseBitMask=off  BitMask=bin2dec('11011001')  BitMaskRealWorld=Stored Integer
  Bitwise_And2 : simulink/Logic and Bit Operations/Bitwise Operator  logicop=AND  UseBitMask=off  BitMask=bin2dec('11011001')  BitMaskRealWorld=Stored Integer
  Bitwise_And3 : simulink/Logic and Bit Operations/Bitwise Operator  logicop=AND  UseBitMask=off  BitMask=bin2dec('11011001')  BitMaskRealWorld=Stored Integer
  Relational Operator : RelationalOperator  Operator===  OutDataTypeStr=boolean  RndMeth=Simplest
  Scope : Scope  NumInputPorts=3
  Scope1 : Scope  NumInputPorts=2
  Scope2 : Scope  NumInputPorts=2
  Scope3 : Scope  NumInputPorts=2
  cmp_2 : UnitTest_Lib/RoughlyEqual  slope=0.1
  cmp_3 : UnitTest_Lib/RoughlyEqual  slope=0.1
  result_tws : ToWorkspace  VariableName=spec_result_003
  tws_1 : ToWorkspace  VariableName=spec_req_003_001
  tws_2 : ToWorkspace  VariableName=spec_req_003_002
  tws_3 : ToWorkspace  VariableName=spec_req_003_003
  result : Outport
  wires:
  sig_Req_Bus/1 -> BS_Req/1
  sig_Result_Bus/1 -> BS_Result/1
  AndN/1 -> result/1, result_tws/1
  BS_Req/1 -> Relational Operator/1, Scope1/1  "<testSig_AirHt_st>"
  BS_Result/1 -> Relational Operator/2, Scope1/2  "<AirHt_st>"
  Relational Operator/1 -> Bitwise_And1/1
  Bitwise_And1/1 -> AndN/1, Scope/1, tws_1/1
  BS_Req/2 -> cmp_2/1, Scope2/1  "<testSig_IAirHt_st>"
  BS_Result/2 -> cmp_2/2, Scope2/2  "<IAirHt_st>"
  cmp_2/1 -> Bitwise_And2/1
  Bitwise_And2/1 -> AndN/2, Scope/2, tws_2/1
  BS_Req/3 -> cmp_3/1, Scope3/1  "<testSig_GlwLmp_st>"
  BS_Result/3 -> cmp_3/2, Scope3/2  "<GlwLmp_st>"
  cmp_3/1 -> Bitwise_And3/1
  Bitwise_And3/1 -> AndN/3, Scope/3, tws_3/1

== system TST_AirHt_Ctl/compareSignals/Requirement_004/specifyOutputs ==
  sig_Req_Bus : Inport
  sig_Result_Bus : Inport  Port=2
  AndN : Logic  Inputs=3
  BS_Req : BusSelector  OutputSignals=testSig_AirHt_st,testSig_IAirHt_st,testSig_GlwLmp_st
  BS_Result : BusSelector  OutputSignals=AirHt_st,IAirHt_st,GlwLmp_st
  Bitwise_And1 : simulink/Logic and Bit Operations/Bitwise Operator  logicop=AND  UseBitMask=off  BitMask=bin2dec('11011001')  BitMaskRealWorld=Stored Integer
  Bitwise_And2 : simulink/Logic and Bit Operations/Bitwise Operator  logicop=AND  UseBitMask=off  BitMask=bin2dec('11011001')  BitMaskRealWorld=Stored Integer
  Bitwise_And3 : simulink/Logic and Bit Operations/Bitwise Operator  logicop=AND  UseBitMask=off  BitMask=bin2dec('11011001')  BitMaskRealWorld=Stored Integer
  Relational Operator : RelationalOperator  Operator===  OutDataTypeStr=boolean  RndMeth=Simplest
  Scope : Scope  NumInputPorts=3
  Scope1 : Scope  NumInputPorts=2
  Scope2 : Scope  NumInputPorts=2
  Scope3 : Scope  NumInputPorts=2
  cmp_2 : UnitTest_Lib/RoughlyEqual  slope=0.1
  cmp_3 : UnitTest_Lib/RoughlyEqual  slope=0.1
  result_tws : ToWorkspace  VariableName=spec_result_004
  tws_1 : ToWorkspace  VariableName=spec_req_004_001
  tws_2 : ToWorkspace  VariableName=spec_req_004_002
  tws_3 : ToWorkspace  VariableName=spec_req_004_003
  result : Outport
  wires:
  sig_Req_Bus/1 -> BS_Req/1
  sig_Result_Bus/1 -> BS_Result/1
  AndN/1 -> result/1, result_tws/1
  BS_Req/1 -> Scope1/1, Relational Operator/1  "<testSig_AirHt_st>"
  BS_Result/1 -> Relational Operator/2, Scope1/2  "<AirHt_st>"
  Relational Operator/1 -> Bitwise_And1/1
  Bitwise_And1/1 -> AndN/1, Scope/1, tws_1/1
  BS_Req/2 -> cmp_2/1, Scope2/1  "<testSig_IAirHt_st>"
  BS_Result/2 -> cmp_2/2, Scope2/2  "<IAirHt_st>"
  cmp_2/1 -> Bitwise_And2/1
  Bitwise_And2/1 -> AndN/2, Scope/2, tws_2/1
  BS_Req/3 -> cmp_3/1, Scope3/1  "<testSig_GlwLmp_st>"
  BS_Result/3 -> cmp_3/2, Scope3/2  "<GlwLmp_st>"
  cmp_3/1 -> Bitwise_And3/1
  Bitwise_And3/1 -> AndN/3, Scope/3, tws_3/1

== system TST_AirHt_Ctl/compareSignals/Requirement_005/specifyOutputs ==
  sig_Req_Bus : Inport
  sig_Result_Bus : Inport  Port=2
  AndN : Logic  Inputs=3
  BS_Req : BusSelector  OutputSignals=testSig_AirHt_st,testSig_IAirHt_st,testSig_GlwLmp_st
  BS_Result : BusSelector  OutputSignals=AirHt_st,IAirHt_st,GlwLmp_st
  Bitwise_And1 : simulink/Logic and Bit Operations/Bitwise Operator  logicop=AND  UseBitMask=off  BitMask=bin2dec('11011001')  BitMaskRealWorld=Stored Integer
  Bitwise_And2 : simulink/Logic and Bit Operations/Bitwise Operator  logicop=AND  UseBitMask=off  BitMask=bin2dec('11011001')  BitMaskRealWorld=Stored Integer
  Bitwise_And3 : simulink/Logic and Bit Operations/Bitwise Operator  logicop=AND  UseBitMask=off  BitMask=bin2dec('11011001')  BitMaskRealWorld=Stored Integer
  Relational Operator : RelationalOperator  Operator===  OutDataTypeStr=boolean  RndMeth=Simplest
  Scope : Scope  NumInputPorts=3
  Scope1 : Scope  NumInputPorts=2
  Scope2 : Scope  NumInputPorts=2
  Scope3 : Scope  NumInputPorts=2
  cmp_2 : UnitTest_Lib/RoughlyEqual  slope=0.1
  cmp_3 : UnitTest_Lib/RoughlyEqual  slope=0.1
  result_tws : ToWorkspace  VariableName=spec_result_005
  tws_1 : ToWorkspace  VariableName=spec_req_005_001
  tws_2 : ToWorkspace  VariableName=spec_req_005_002
  tws_3 : ToWorkspace  VariableName=spec_req_005_003
  result : Outport
  wires:
  sig_Req_Bus/1 -> BS_Req/1
  sig_Result_Bus/1 -> BS_Result/1
  AndN/1 -> result/1, result_tws/1
  BS_Req/1 -> Relational Operator/1, Scope1/1  "<testSig_AirHt_st>"
  BS_Result/1 -> Relational Operator/2, Scope1/2  "<AirHt_st>"
  Relational Operator/1 -> Bitwise_And1/1
  Bitwise_And1/1 -> AndN/1, Scope/1, tws_1/1
  BS_Req/2 -> cmp_2/1, Scope2/1  "<testSig_IAirHt_st>"
  BS_Result/2 -> cmp_2/2, Scope2/2  "<IAirHt_st>"
  cmp_2/1 -> Bitwise_And2/1
  Bitwise_And2/1 -> AndN/2, Scope/2, tws_2/1
  BS_Req/3 -> cmp_3/1, Scope3/1  "<testSig_GlwLmp_st>"
  BS_Result/3 -> cmp_3/2, Scope3/2  "<GlwLmp_st>"
  cmp_3/1 -> Bitwise_And3/1
  Bitwise_And3/1 -> AndN/3, Scope/3, tws_3/1

== system TST_AirHt_Ctl/compareSignals/Requirement_006/specifyOutputs ==
  sig_Req_Bus : Inport
  sig_Result_Bus : Inport  Port=2
  AndN : Logic  Inputs=3
  BS_Req : BusSelector  OutputSignals=testSig_AirHt_st,testSig_IAirHt_st,testSig_GlwLmp_st
  BS_Result : BusSelector  OutputSignals=AirHt_st,IAirHt_st,GlwLmp_st
  Bitwise_And1 : simulink/Logic and Bit Operations/Bitwise Operator  logicop=AND  UseBitMask=off  BitMask=bin2dec('11011001')  BitMaskRealWorld=Stored Integer
  Bitwise_And2 : simulink/Logic and Bit Operations/Bitwise Operator  logicop=AND  UseBitMask=off  BitMask=bin2dec('11011001')  BitMaskRealWorld=Stored Integer
  Bitwise_And3 : simulink/Logic and Bit Operations/Bitwise Operator  logicop=AND  UseBitMask=off  BitMask=bin2dec('11011001')  BitMaskRealWorld=Stored Integer
  Relational Operator : RelationalOperator  Operator===  OutDataTypeStr=boolean  RndMeth=Simplest
  Scope : Scope  NumInputPorts=3
  Scope1 : Scope  NumInputPorts=2
  Scope2 : Scope  NumInputPorts=2
  Scope3 : Scope  NumInputPorts=2
  cmp_2 : UnitTest_Lib/RoughlyEqual  slope=0.1
  cmp_3 : UnitTest_Lib/RoughlyEqual  slope=0.1
  result_tws : ToWorkspace  VariableName=spec_result_006
  tws_1 : ToWorkspace  VariableName=spec_req_006_001
  tws_2 : ToWorkspace  VariableName=spec_req_006_002
  tws_3 : ToWorkspace  VariableName=spec_req_006_003
  result : Outport
  wires:
  sig_Req_Bus/1 -> BS_Req/1
  sig_Result_Bus/1 -> BS_Result/1
  AndN/1 -> result/1, result_tws/1
  BS_Req/1 -> Relational Operator/1, Scope1/1  "<testSig_AirHt_st>"
  BS_Result/1 -> Relational Operator/2, Scope1/2  "<AirHt_st>"
  Relational Operator/1 -> Bitwise_And1/1
  Bitwise_And1/1 -> AndN/1, Scope/1, tws_1/1
  BS_Req/2 -> cmp_2/1, Scope2/1  "<testSig_IAirHt_st>"
  BS_Result/2 -> cmp_2/2, Scope2/2  "<IAirHt_st>"
  cmp_2/1 -> Bitwise_And2/1
  Bitwise_And2/1 -> AndN/2, Scope/2, tws_2/1
  BS_Req/3 -> cmp_3/1, Scope3/1  "<testSig_GlwLmp_st>"
  BS_Result/3 -> cmp_3/2, Scope3/2  "<GlwLmp_st>"
  cmp_3/1 -> Bitwise_And3/1
  Bitwise_And3/1 -> AndN/3, Scope/3, tws_3/1

== system TST_AirHt_Ctl/compareSignals/Requirement_007/specifyOutputs ==
  sig_Req_Bus : Inport
  sig_Result_Bus : Inport  Port=2
  AndN : Logic  Inputs=3
  BS_Req : BusSelector  OutputSignals=testSig_AirHt_st,testSig_IAirHt_st,testSig_GlwLmp_st
  BS_Result : BusSelector  OutputSignals=AirHt_st,IAirHt_st,GlwLmp_st
  Bitwise_And1 : simulink/Logic and Bit Operations/Bitwise Operator  logicop=AND  UseBitMask=off  BitMask=bin2dec('11011001')  BitMaskRealWorld=Stored Integer
  Bitwise_And2 : simulink/Logic and Bit Operations/Bitwise Operator  logicop=AND  UseBitMask=off  BitMask=bin2dec('11011001')  BitMaskRealWorld=Stored Integer
  Bitwise_And3 : simulink/Logic and Bit Operations/Bitwise Operator  logicop=AND  UseBitMask=off  BitMask=bin2dec('11011001')  BitMaskRealWorld=Stored Integer
  Relational Operator : RelationalOperator  Operator===  OutDataTypeStr=boolean  RndMeth=Simplest
  Scope : Scope  NumInputPorts=3
  Scope1 : Scope  NumInputPorts=2
  Scope2 : Scope  NumInputPorts=2
  Scope3 : Scope  NumInputPorts=2
  cmp_2 : UnitTest_Lib/RoughlyEqual  slope=0.1
  cmp_3 : UnitTest_Lib/RoughlyEqual  slope=0.1
  result_tws : ToWorkspace  VariableName=spec_result_007
  tws_1 : ToWorkspace  VariableName=spec_req_007_001
  tws_2 : ToWorkspace  VariableName=spec_req_007_002
  tws_3 : ToWorkspace  VariableName=spec_req_007_003
  result : Outport
  wires:
  sig_Req_Bus/1 -> BS_Req/1
  sig_Result_Bus/1 -> BS_Result/1
  AndN/1 -> result/1, result_tws/1
  BS_Req/1 -> Scope1/1, Relational Operator/1  "<testSig_AirHt_st>"
  BS_Result/1 -> Relational Operator/2, Scope1/2  "<AirHt_st>"
  Relational Operator/1 -> Bitwise_And1/1
  Bitwise_And1/1 -> AndN/1, Scope/1, tws_1/1
  BS_Req/2 -> cmp_2/1, Scope2/1  "<testSig_IAirHt_st>"
  BS_Result/2 -> cmp_2/2, Scope2/2  "<IAirHt_st>"
  cmp_2/1 -> Bitwise_And2/1
  Bitwise_And2/1 -> AndN/2, Scope/2, tws_2/1
  BS_Req/3 -> cmp_3/1, Scope3/1  "<testSig_GlwLmp_st>"
  BS_Result/3 -> cmp_3/2, Scope3/2  "<GlwLmp_st>"
  cmp_3/1 -> Bitwise_And3/1
  Bitwise_And3/1 -> AndN/3, Scope/3, tws_3/1

== system TST_AirHt_Ctl/compareSignals/Requirement_008/specifyOutputs ==
  sig_Req_Bus : Inport
  sig_Result_Bus : Inport  Port=2
  AndN : Logic  Inputs=3
  BS_Req : BusSelector  OutputSignals=testSig_AirHt_st,testSig_IAirHt_st,testSig_GlwLmp_st
  BS_Result : BusSelector  OutputSignals=AirHt_st,IAirHt_st,GlwLmp_st
  Bitwise_And1 : simulink/Logic and Bit Operations/Bitwise Operator  logicop=AND  UseBitMask=off  BitMask=bin2dec('11011001')  BitMaskRealWorld=Stored Integer
  Bitwise_And2 : simulink/Logic and Bit Operations/Bitwise Operator  logicop=AND  UseBitMask=off  BitMask=bin2dec('11011001')  BitMaskRealWorld=Stored Integer
  Bitwise_And3 : simulink/Logic and Bit Operations/Bitwise Operator  logicop=AND  UseBitMask=off  BitMask=bin2dec('11011001')  BitMaskRealWorld=Stored Integer
  Relational Operator : RelationalOperator  Operator===  OutDataTypeStr=boolean  RndMeth=Simplest
  Scope : Scope  NumInputPorts=3
  Scope1 : Scope  NumInputPorts=2
  Scope2 : Scope  NumInputPorts=2
  Scope3 : Scope  NumInputPorts=2
  cmp_2 : UnitTest_Lib/RoughlyEqual  slope=0.1
  cmp_3 : UnitTest_Lib/RoughlyEqual  slope=0.1
  result_tws : ToWorkspace  VariableName=spec_result_008
  tws_1 : ToWorkspace  VariableName=spec_req_008_001
  tws_2 : ToWorkspace  VariableName=spec_req_008_002
  tws_3 : ToWorkspace  VariableName=spec_req_008_003
  result : Outport
  wires:
  sig_Req_Bus/1 -> BS_Req/1
  sig_Result_Bus/1 -> BS_Result/1
  AndN/1 -> result/1, result_tws/1
  BS_Req/1 -> Relational Operator/1, Scope1/1  "<testSig_AirHt_st>"
  BS_Result/1 -> Relational Operator/2, Scope1/2  "<AirHt_st>"
  Relational Operator/1 -> Bitwise_And1/1
  Bitwise_And1/1 -> AndN/1, Scope/1, tws_1/1
  BS_Req/2 -> cmp_2/1, Scope2/1  "<testSig_IAirHt_st>"
  BS_Result/2 -> cmp_2/2, Scope2/2  "<IAirHt_st>"
  cmp_2/1 -> Bitwise_And2/1
  Bitwise_And2/1 -> AndN/2, Scope/2, tws_2/1
  BS_Req/3 -> cmp_3/1, Scope3/1  "<testSig_GlwLmp_st>"
  BS_Result/3 -> cmp_3/2, Scope3/2  "<GlwLmp_st>"
  cmp_3/1 -> Bitwise_And3/1
  Bitwise_And3/1 -> AndN/3, Scope/3, tws_3/1
